simulink model "elcentro_NS"  (R2015b)
settings: Solver=VariableStepAuto  StartTime=0.0  StopTime=50  RelTol=1e-3
undefined symbols (not defined in the file or in its folder): DiscIntNeverNeededParam, get, sigbuilder_block
libraries: dspxfrm3 x1, dspsnks4 x1
settings Model: Creator=YogurtSuee  LastModifiedBy=YogurtSuee

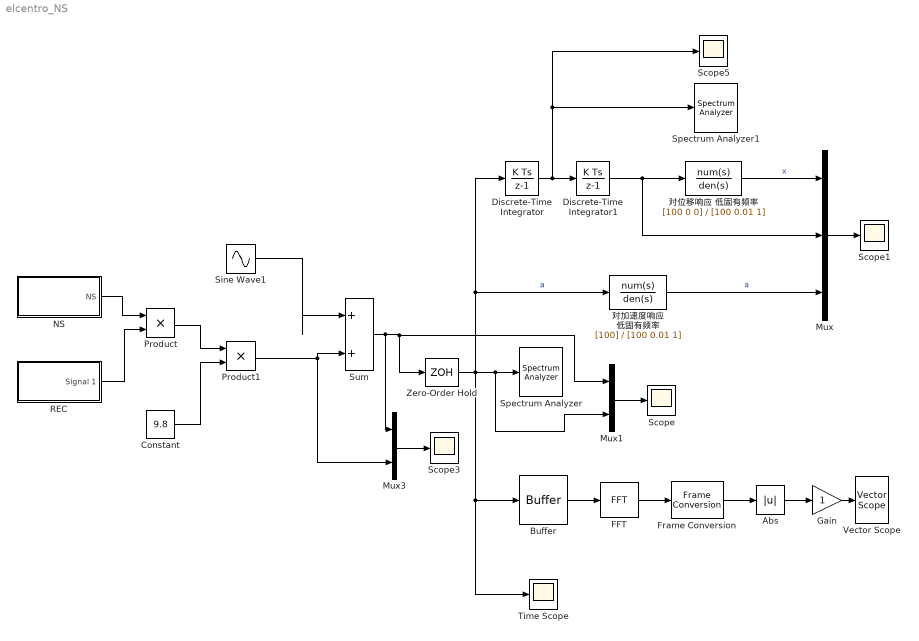
== system elcentro_NS ==
  Abs : Abs
  Buffer : Buffer  N=256  TreatMby1Signals=One channel  OutputFrames=off
  Constant : Constant  Value=9.8
  Discrete-Time Integrator : DiscreteIntegrator  InitialConditionSetting=State (most efficient)  SampleTime=0.02  ICPrevOutput=DiscIntNeverNeededParam  ICPrevScaledInput=DiscIntNeverNeededParam
  Discrete-Time Integrator1 : DiscreteIntegrator  InitialConditionSetting=State (most efficient)  SampleTime=0.02  ICPrevOutput=DiscIntNeverNeededParam  ICPrevScaledInput=DiscIntNeverNeededParam
  FFT : dspxfrm3/FFT  FFTImplementation=Auto  CompMethod=Table lookup  TableOpt=NEW  TableOptActive=Speed  BitRevOrder=off  Normalize=off  InheritFFTLength=on  FFTLength=64  WrapInput=on  roundingMode=Floor  overflowMode=off  firstCoeffDataTypeStr=Inherit: Same word length as input  firstCoeffLastDataTypeStr=Inherit: Same word length as input  outputMin=[]  outputMax=[]
  Frame Conversion : FrameConversion  InheritSamplingMode=off
  Gain : Gain
  Mux : Mux  Inputs=3
  Mux1 : Mux  Inputs=2
  Mux3 : Mux  Inputs=2
  NS : Subsystem  Tag=STV Subsys  LoadFcn=sigbuilder_block('load');  StartFcn=sigbuilder_block('start');  StopFcn=sigbuilder_block('stop');  ClipboardFcn=sigbuilder_block('clipboard');  mask(Sigbuilder block){}
      mask help: Simulink:masks:SigbuilderBlock_MD
      mask init:
      | if ~strcmp(get_param(bdroot(gcbh),'SimulationStatus'),'stopped') tuvar = sigbuilder_block('maskInit'); end
      settings: CopyFcn=sigbuilder_block('copy');  DeleteFcn=sigbuilder_block('delete');  ModelCloseFcn=sigbuilder_block('modelClose');  PreSaveFcn=sigbuilder_block('preSave');  PauseFcn=sigbuilder_block('pause');  ContinueFcn=sigbuilder_block('continue');  NameChangeFcn=sigbuilder_block('namechange');  OpenFcn=sigbuilder_block('open',[437.6 199.2 550.4 400 ]);  CloseFcn=sigbuilder_block('close');
      mask Display: plot(0, 0, 100, 100,[2, 2, 32, 32, 2], [68, 8, 8, 68, 68],[32, 2], [38, 38], [32, 19, 2],[53, 60, 44], [32, 17, 17, 2],[16, 16, 31, 31]);txt = getActiveGroup(gcbh);text(2, 100, txt,'verticalAlignment', 'top');
  Product : Product
  Product1 : Product
  REC : Subsystem  Tag=STV Subsys  LoadFcn=sigbuilder_block('load');  StartFcn=sigbuilder_block('start');  StopFcn=sigbuilder_block('stop');  ClipboardFcn=sigbuilder_block('clipboard');  mask(Sigbuilder block){}
      mask help: Simulink:masks:SigbuilderBlock_MD
      mask init:
      | if ~strcmp(get_param(bdroot(gcbh),'SimulationStatus'),'stopped') tuvar = sigbuilder_block('maskInit'); end
      settings: CopyFcn=sigbuilder_block('copy');  DeleteFcn=sigbuilder_block('delete');  ModelCloseFcn=sigbuilder_block('modelClose');  PreSaveFcn=sigbuilder_block('preSave');  PauseFcn=sigbuilder_block('pause');  ContinueFcn=sigbuilder_block('continue');  NameChangeFcn=sigbuilder_block('namechange');  OpenFcn=sigbuilder_block('open',[437.6 199.2 550.4 400 ]);  CloseFcn=sigbuilder_block('close');
      mask Display: plot(0, 0, 100, 100,[2, 2, 32, 32, 2], [68, 8, 8, 68, 68],[32, 2], [38, 38], [32, 19, 2],[53, 60, 44], [32, 17, 17, 2],[16, 16, 31, 31]);txt = getActiveGroup(gcbh);text(2, 100, txt,'verticalAlignment', 'top');
  Scope{,1,3,5} (4 alike) : Scope
  Sine Wave1 : Sin  Amplitude=2  Frequency=20  SampleTime=0
  Spectrum Analyzer : SpectrumAnalyzer
  Spectrum Analyzer1 : SpectrumAnalyzer
  Sum : Sum  Inputs=|++
  Time Scope : Scope
  Vector Scope : dspsnks4/Vector Scope  ScopeProperties=on  Domain=Frequency  HorizSpan=1  DisplayProperties=off  AxisGrid=on  Memory=off  FrameNumber=on  AxisLegend=off  AxisZoom=on  OpenScopeAtSimStart=on  OpenScopeImmediately=off  FigPos=get(0,'defaultfigureposition')  AxisProperties=off  XUnits=Hertz  XRange=[0...Fs/2]  InheritXIncr=on  XIncr=1  XLabel=Time  XLimit=Auto  XMin=0  XMax=1  XStart=0  YUnits=Magnitude  YLabel=Amplitude  LineProperties=off  LineMarkers=+  XAxisParamsVer=6.9
      settings: YMin=-2  YMax=60
  Zero-Order Hold : ZeroOrderHold  SampleTime=0.02
  对位移响应 低固有频率 : TransferFcn  Numerator=[100 0 0]  Denominator=[100 0.01 1]
  对加速度响应 低固有频率 : TransferFcn  Numerator=[100]  Denominator=[100 0.01 1]
  wires:
  Product/1 -> Product1/1
  NS/1(NS) -> Product/1
  REC/1(Signal 1) -> Product/2
  Constant/1 -> Product1/2
  Zero-Order Hold/1 -> Discrete-Time Integrator/1, 对加速度响应 低固有频率/1, Time Scope/1, Buffer/1, Mux1/2, Spectrum Analyzer/1  "a"
  Buffer/1 -> FFT/1
  FFT/1 -> Frame Conversion/1
  Frame Conversion/1 -> Abs/1
  Abs/1 -> Gain/1
  Gain/1 -> Vector Scope/1
  Mux/1 -> Scope1/1
  对位移响应 低固有频率/1 -> Mux/1  "x"
  Discrete-Time Integrator/1 -> Scope5/1, Spectrum Analyzer1/1, Discrete-Time Integrator1/1
  Discrete-Time Integrator1/1 -> Mux/2, 对位移响应 低固有频率/1
  对加速度响应 低固有频率/1 -> Mux/3  "a"
  Mux1/1 -> Scope/1
  Sine Wave1/1 -> Sum/1
  Sum/1 -> Mux3/1, Mux1/1, Zero-Order Hold/1
  Product1/1 -> Mux3/2, Sum/2
  Mux3/1 -> Scope3/1

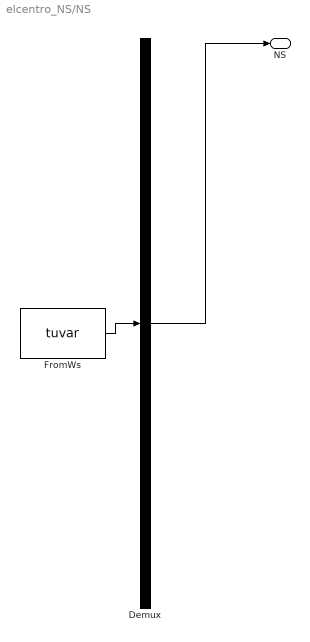
== system elcentro_NS/NS ==
  Demux : Demux  Tag=STV Demux  Outputs=1
  FromWs : FromWorkspace  Tag=STV FromWs  VariableName=tuvar  SampleTime=0
      SigBuilderData=|
      | common.afterFinalStr = 'Extrapolate'
      | common.sampleTime = 0
      | dataSet.timeRange = [0 53.74]
      | dataSet.name = '南北方向'
      | sbobj.Name = 'Signal Builder'
      | sbobj.Groups.Name = '南北方向'
      | sbobj.Groups.Signals.Name = 'NS'
      | sbobj.Groups.Signals.XData = [0 0.02 0.04 0.06 0.08 0.1 0.12 0.14 0.16 0.18 0.2 0.22 ... (2688 elements, 1x2688)]
      | sbobj.Groups.Signals.YData = [-0.0014275799 -0.01101276 -0.01029897 -0.0089733599 -0.0096871497 -0.0122364 -0.014479739 -0.01305216 -0.0112167 -0.0086674497 -0.0086674497 -0.01335807 ... (2688 elements, 1x2688)]
      | sbobj.Groups.TimeRange = [0 53.74]
  NS : Outport
  wires:
  Demux/1 -> NS/1
  FromWs/1 -> Demux/1

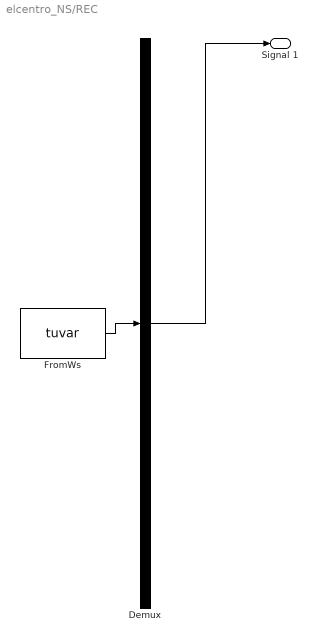
== system elcentro_NS/REC ==
  Demux : Demux  Tag=STV Demux  Outputs=1
  FromWs : FromWorkspace  Tag=STV FromWs  VariableName=tuvar  SampleTime=0
      SigBuilderData=|
      | common.afterFinalStr = 'Extrapolate'
      | common.sampleTime = 0
      | dataSet.timeRange = [0 60]
      | dataSet.name = 'Group 1'
      | sbobj.Groups.Name = 'Group 1'
      | sbobj.Groups.Signals.Name = 'Signal 1'
      | sbobj.Groups.Signals.XData = [0 50 50 60]
      | sbobj.Groups.Signals.YData = [1 1 0 0]
      | sbobj.Groups.TimeRange = [0 60]
  Signal 1 : Outport  Tag=STV Outport
  wires:
  Demux/1 -> Signal 1/1
  FromWs/1 -> Demux/1
